simulink model "only_plant"  (R2018b)
settings: Solver=VariableStepAuto  StartTime=0.0  StopTime=10  FixedStep=0.02  RelTol=1e-3  EnableMultiTasking=on
values from neighbouring files (symbols this model uses):
  Kp = 10    [init_transfers_knut.m]
  R = 0.08    [init_transfers_knut.m]
  Td = 0    [init_transfers_knut.m]
  Tf = 0.05    [init_transfers_knut.m]
  Ti = 9.1    [init_transfers_knut.m]
  Ty = 0.2    [init_transfers_knut.m]
  Ysp = 0    [init_transfers_knut.m]
undefined symbols (not defined in the file or in its folder): Tw
settings Model: Creator=sigurdj  LastModifiedBy=sigurd
settings DataIOCC: LimitDataPoints=on  SaveFormat=Array
settings OptimizationCC: LifeSpan=inf
settings DebuggingCC: SolverPrmCheckMsg=warning  SFUnexpectedBacktrackingDiag=warning  SFNoUnconditionalDefaultTransitionDiag=warning
settings HardwareCC: ProdBitPerPointer=32  ProdBitPerSizeT=32  ProdBitPerPtrDiffT=32  ProdLargestAtomicFloat=None  ProdIntDivRoundTo=Undefined  ProdEndianess=Unspecified  ProdWordSize=32  ProdHWDeviceType=32-bit Generic
settings ModelReferenceCC: PropagateSignalLabelsOutOfModel=off
settings SFSimCC: SimUseLocalCustomCode=off
settings RTWCC: RTWUseLocalCustomCode=off
settings CodeAppCC: StateflowObjectComments=on
settings GRTTargetCC: TargetLangStandard=C89/C90 (ANSI)  GeneratePreprocessorConditionals=Disable all
settings ConfigComp: CovMetricSettings=dw  CovHtmlReporting=on  CovSaveCumulativeToWorkspaceVar=on  CovSaveSingleToWorkspaceVar=on  CovExternalEMLEnable=off  CovSFcnEnable=off

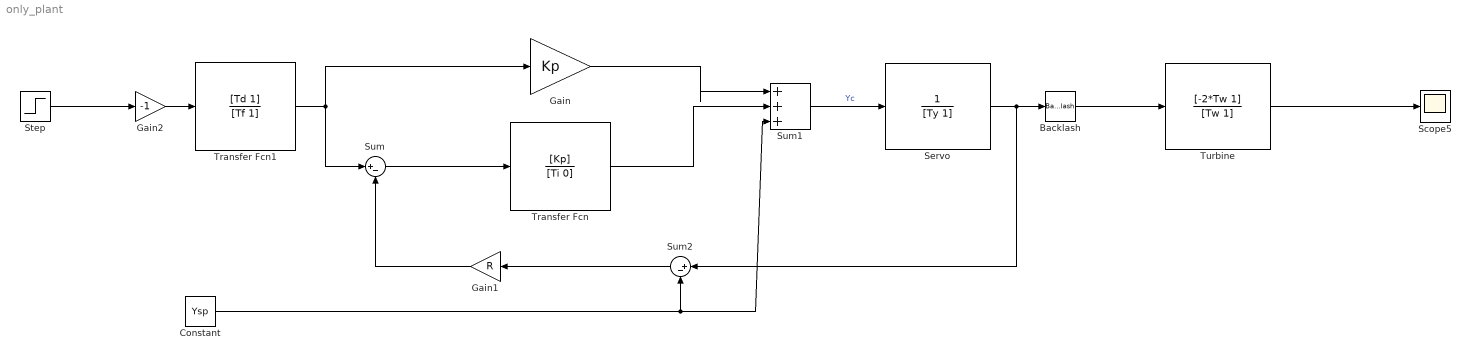
== system only_plant ==
  Backlash : Backlash  BacklashWidth=Ksp
  Constant : Constant  Value=Ysp
  Gain : Gain  Gain=Kp
  Gain1 : Gain  Gain=R
  Gain2 : Gain  Gain=-1
  Scope5 : Scope
  Servo : TransferFcn  Denominator=[Ty 1]
  Step : Step  SampleTime=0
  Sum : Sum  Inputs=|+-
  Sum1 : Sum  Inputs=|+++
  Sum2 : Sum  Inputs=|+-
  Transfer Fcn : TransferFcn  Numerator=[Kp]  Denominator=[Ti 0]
  Transfer Fcn1 : TransferFcn  Numerator=[Td 1]  Denominator=[Tf 1]
  Turbine : TransferFcn  Numerator=[-2*Tw 1]  Denominator=[Tw 1]
  wires:
  Turbine/1 -> Scope5/1
  Step/1 -> Gain2/1
  Transfer Fcn1/1 -> Gain/1, Sum/1
  Sum2/1 -> Gain1/1
  Gain1/1 -> Sum/2
  Constant/1 -> Sum1/3, Sum2/2
  Servo/1 -> Backlash/1, Sum2/1
  Gain/1 -> Sum1/1
  Gain2/1 -> Transfer Fcn1/1
  Sum1/1 -> Servo/1  "Yc"
  Sum/1 -> Transfer Fcn/1
  Transfer Fcn/1 -> Sum1/2
  Backlash/1 -> Turbine/1
